simulink model "TST_PIntkVUs_DD"  (R2016b)
settings: Solver=FixedStepDiscrete  StartTime=0.0  StopTime=simTime  FixedStep=sampleTime  RelTol=1e-3
values from neighbouring files (symbols this model uses):
  testCase = 1    [initTST_PIntkVUs_DD_001.m]    (also in initTST_PIntkVUs_DD_002.m = 2; initTST_PIntkVUs_DD_003.m = 3; initTST_PIntkVUs_DD_004.m = 4; initTST_PIntkVUs_DD_005.m = 5)
libraries: UnitTest_Lib x98, simulink x8
(part 2 of 3)

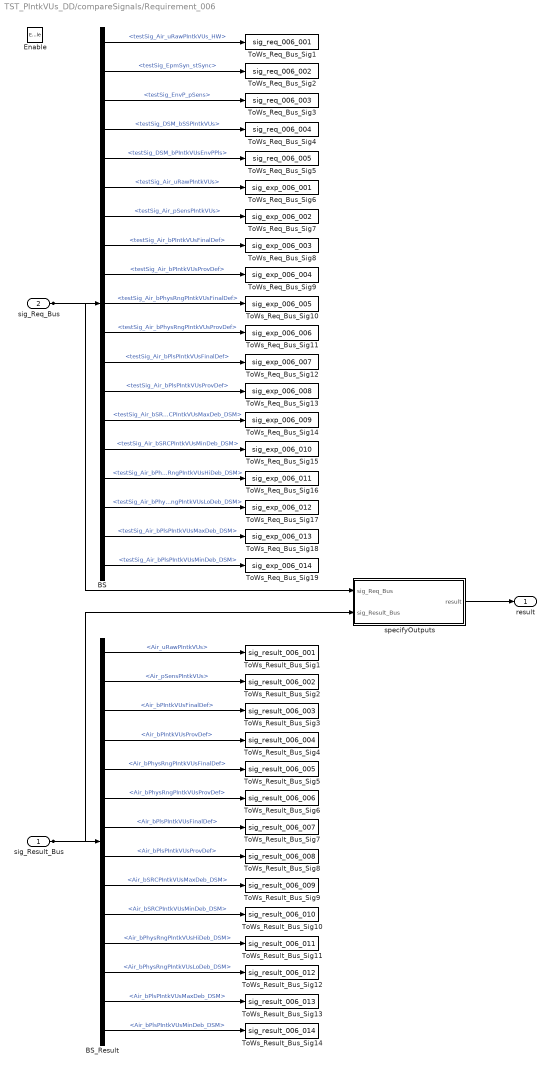
== system TST_PIntkVUs_DD/compareSignals/Requirement_006 ==
  sig_Result_Bus : Inport
  sig_Req_Bus : Inport  Port=2
  Enable : EnablePort
  BS : BusSelector  OutputSignals=testSig_Air_uRawPIntkVUs_HW,testSig_EpmSyn_stSync,testSig_EnvP_pSens,testSig_DSM_bSSPIntkVUs,testSig_DSM_bPIntkVUsEnvPPls,testSig_Air_uRawPIntkVUs,testSig_Air_pSensPIntkVUs,testSig_Air_bPIntkVUsFinalDef,testSig_Air_bPIntkVUsProvDef,testSig_Air_bPhysRngPIntkVUsFinalDef,testSig_Air_bPhysRngPIntkVUsProvDef,testSig_Air_bPlsPIntkVUsFinalDef,testSig_Air_bPlsPIntkVUsProvDef,testSig_Air_bSRCPIntkVUsMaxDeb_DSM,testSig_Air_bSRCPIntkVUsMinDeb_DSM,testSig_Air_bPhysRngPIntkVUsHiDeb_DSM,testSig_Air_bPhysRngPIntkVUsLoDeb_DSM,testSig_Air_bPlsPIntkVUsMaxDeb_DSM,testSig_Air_bPlsPIntkVUsMinDeb_DSM
  BS_Result : BusSelector  OutputSignals=Air_uRawPIntkVUs,Air_pSensPIntkVUs,Air_bPIntkVUsFinalDef,Air_bPIntkVUsProvDef,Air_bPhysRngPIntkVUsFinalDef,Air_bPhysRngPIntkVUsProvDef,Air_bPlsPIntkVUsFinalDef,Air_bPlsPIntkVUsProvDef,Air_bSRCPIntkVUsMaxDeb_DSM,Air_bSRCPIntkVUsMinDeb_DSM,Air_bPhysRngPIntkVUsHiDeb_DSM,Air_bPhysRngPIntkVUsLoDeb_DSM,Air_bPlsPIntkVUsMaxDeb_DSM,Air_bPlsPIntkVUsMinDeb_DSM
  ToWs_Req_Bus_Sig1 : ToWorkspace  VariableName=sig_req_006_001  SaveFormat=Structure With Time
  ToWs_Req_Bus_Sig10 : ToWorkspace  VariableName=sig_exp_006_005  SaveFormat=Structure With Time
  ToWs_Req_Bus_Sig11 : ToWorkspace  VariableName=sig_exp_006_006  SaveFormat=Structure With Time
  ToWs_Req_Bus_Sig12 : ToWorkspace  VariableName=sig_exp_006_007  SaveFormat=Structure With Time
  ToWs_Req_Bus_Sig13 : ToWorkspace  VariableName=sig_exp_006_008  SaveFormat=Structure With Time
  ToWs_Req_Bus_Sig14 : ToWorkspace  VariableName=sig_exp_006_009  SaveFormat=Structure With Time
  ToWs_Req_Bus_Sig15 : ToWorkspace  VariableName=sig_exp_006_010  SaveFormat=Structure With Time
  ToWs_Req_Bus_Sig16 : ToWorkspace  VariableName=sig_exp_006_011  SaveFormat=Structure With Time
  ToWs_Req_Bus_Sig17 : ToWorkspace  VariableName=sig_exp_006_012  SaveFormat=Structure With Time
  ToWs_Req_Bus_Sig18 : ToWorkspace  VariableName=sig_exp_006_013  SaveFormat=Structure With Time
  ToWs_Req_Bus_Sig19 : ToWorkspace  VariableName=sig_exp_006_014  SaveFormat=Structure With Time
  ToWs_Req_Bus_Sig2 : ToWorkspace  VariableName=sig_req_006_002  SaveFormat=Structure With Time
  ToWs_Req_Bus_Sig3 : ToWorkspace  VariableName=sig_req_006_003  SaveFormat=Structure With Time
  ToWs_Req_Bus_Sig4 : ToWorkspace  VariableName=sig_req_006_004  SaveFormat=Structure With Time
  ToWs_Req_Bus_Sig5 : ToWorkspace  VariableName=sig_req_006_005  SaveFormat=Structure With Time
  ToWs_Req_Bus_Sig6 : ToWorkspace  VariableName=sig_exp_006_001  SaveFormat=Structure With Time
  ToWs_Req_Bus_Sig7 : ToWorkspace  VariableName=sig_exp_006_002  SaveFormat=Structure With Time
  ToWs_Req_Bus_Sig8 : ToWorkspace  VariableName=sig_exp_006_003  SaveFormat=Structure With Time
  ToWs_Req_Bus_Sig9 : ToWorkspace  VariableName=sig_exp_006_004  SaveFormat=Structure With Time
  ToWs_Result_Bus_Sig1 : ToWorkspace  VariableName=sig_result_006_001  SaveFormat=Structure With Time
  ToWs_Result_Bus_Sig10 : ToWorkspace  VariableName=sig_result_006_010  SaveFormat=Structure With Time
  ToWs_Result_Bus_Sig11 : ToWorkspace  VariableName=sig_result_006_011  SaveFormat=Structure With Time
  ToWs_Result_Bus_Sig12 : ToWorkspace  VariableName=sig_result_006_012  SaveFormat=Structure With Time
  ToWs_Result_Bus_Sig13 : ToWorkspace  VariableName=sig_result_006_013  SaveFormat=Structure With Time
  ToWs_Result_Bus_Sig14 : ToWorkspace  VariableName=sig_result_006_014  SaveFormat=Structure With Time
  ToWs_Result_Bus_Sig2 : ToWorkspace  VariableName=sig_result_006_002  SaveFormat=Structure With Time
  ToWs_Result_Bus_Sig3 : ToWorkspace  VariableName=sig_result_006_003  SaveFormat=Structure With Time
  ToWs_Result_Bus_Sig4 : ToWorkspace  VariableName=sig_result_006_004  SaveFormat=Structure With Time
  ToWs_Result_Bus_Sig5 : ToWorkspace  VariableName=sig_result_006_005  SaveFormat=Structure With Time
  ToWs_Result_Bus_Sig6 : ToWorkspace  VariableName=sig_result_006_006  SaveFormat=Structure With Time
  ToWs_Result_Bus_Sig7 : ToWorkspace  VariableName=sig_result_006_007  SaveFormat=Structure With Time
  ToWs_Result_Bus_Sig8 : ToWorkspace  VariableName=sig_result_006_008  SaveFormat=Structure With Time
  ToWs_Result_Bus_Sig9 : ToWorkspace  VariableName=sig_result_006_009  SaveFormat=Structure With Time
  specifyOutputs : Subsystem
  result : Outport
  wires:
  sig_Req_Bus/1 -> BS/1, specifyOutputs/1(sig_Req_Bus)
  BS/1 -> ToWs_Req_Bus_Sig1/1  "<testSig_Air_uRawPIntkVUs_HW>"
  BS/2 -> ToWs_Req_Bus_Sig2/1  "<testSig_EpmSyn_stSync>"
  BS/3 -> ToWs_Req_Bus_Sig3/1  "<testSig_EnvP_pSens>"
  BS/4 -> ToWs_Req_Bus_Sig4/1  "<testSig_DSM_bSSPIntkVUs>"
  BS/5 -> ToWs_Req_Bus_Sig5/1  "<testSig_DSM_bPIntkVUsEnvPPls>"
  BS/6 -> ToWs_Req_Bus_Sig6/1  "<testSig_Air_uRawPIntkVUs>"
  BS/7 -> ToWs_Req_Bus_Sig7/1  "<testSig_Air_pSensPIntkVUs>"
  BS/8 -> ToWs_Req_Bus_Sig8/1  "<testSig_Air_bPIntkVUsFinalDef>"
  BS/9 -> ToWs_Req_Bus_Sig9/1  "<testSig_Air_bPIntkVUsProvDef>"
  BS/10 -> ToWs_Req_Bus_Sig10/1  "<testSig_Air_bPhysRngPIntkVUsFinalDef>"
  BS/11 -> ToWs_Req_Bus_Sig11/1  "<testSig_Air_bPhysRngPIntkVUsProvDef>"
  BS/12 -> ToWs_Req_Bus_Sig12/1  "<testSig_Air_bPlsPIntkVUsFinalDef>"
  BS/13 -> ToWs_Req_Bus_Sig13/1  "<testSig_Air_bPlsPIntkVUsProvDef>"
  BS/14 -> ToWs_Req_Bus_Sig14/1  "<testSig_Air_bSRCPIntkVUsMaxDeb_DSM>"
  BS/15 -> ToWs_Req_Bus_Sig15/1  "<testSig_Air_bSRCPIntkVUsMinDeb_DSM>"
  BS/16 -> ToWs_Req_Bus_Sig16/1  "<testSig_Air_bPhysRngPIntkVUsHiDeb_DSM>"
  BS/17 -> ToWs_Req_Bus_Sig17/1  "<testSig_Air_bPhysRngPIntkVUsLoDeb_DSM>"
  BS/18 -> ToWs_Req_Bus_Sig18/1  "<testSig_Air_bPlsPIntkVUsMaxDeb_DSM>"
  BS/19 -> ToWs_Req_Bus_Sig19/1  "<testSig_Air_bPlsPIntkVUsMinDeb_DSM>"
  sig_Result_Bus/1 -> BS_Result/1, specifyOutputs/2(sig_Result_Bus)
  BS_Result/1 -> ToWs_Result_Bus_Sig1/1  "<Air_uRawPIntkVUs>"
  BS_Result/2 -> ToWs_Result_Bus_Sig2/1  "<Air_pSensPIntkVUs>"
  BS_Result/3 -> ToWs_Result_Bus_Sig3/1  "<Air_bPIntkVUsFinalDef>"
  BS_Result/4 -> ToWs_Result_Bus_Sig4/1  "<Air_bPIntkVUsProvDef>"
  BS_Result/5 -> ToWs_Result_Bus_Sig5/1  "<Air_bPhysRngPIntkVUsFinalDef>"
  BS_Result/6 -> ToWs_Result_Bus_Sig6/1  "<Air_bPhysRngPIntkVUsProvDef>"
  BS_Result/7 -> ToWs_Result_Bus_Sig7/1  "<Air_bPlsPIntkVUsFinalDef>"
  BS_Result/8 -> ToWs_Result_Bus_Sig8/1  "<Air_bPlsPIntkVUsProvDef>"
  BS_Result/9 -> ToWs_Result_Bus_Sig9/1  "<Air_bSRCPIntkVUsMaxDeb_DSM>"
  BS_Result/10 -> ToWs_Result_Bus_Sig10/1  "<Air_bSRCPIntkVUsMinDeb_DSM>"
  BS_Result/11 -> ToWs_Result_Bus_Sig11/1  "<Air_bPhysRngPIntkVUsHiDeb_DSM>"
  BS_Result/12 -> ToWs_Result_Bus_Sig12/1  "<Air_bPhysRngPIntkVUsLoDeb_DSM>"
  BS_Result/13 -> ToWs_Result_Bus_Sig13/1  "<Air_bPlsPIntkVUsMaxDeb_DSM>"
  BS_Result/14 -> ToWs_Result_Bus_Sig14/1  "<Air_bPlsPIntkVUsMinDeb_DSM>"
  specifyOutputs/1(result) -> result/1

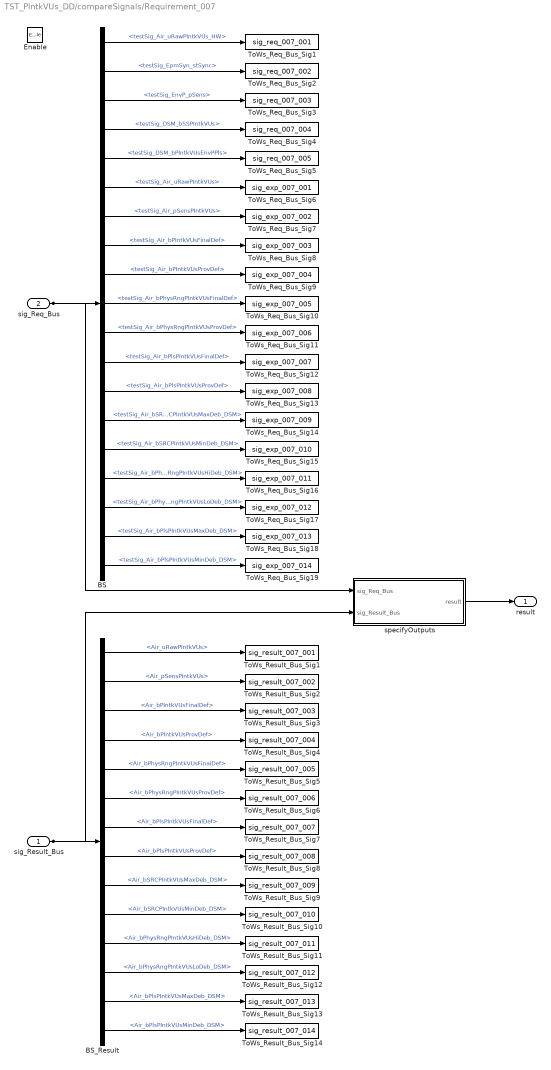
== system TST_PIntkVUs_DD/compareSignals/Requirement_007 ==
  sig_Result_Bus : Inport
  sig_Req_Bus : Inport  Port=2
  Enable : EnablePort
  BS : BusSelector  OutputSignals=testSig_Air_uRawPIntkVUs_HW,testSig_EpmSyn_stSync,testSig_EnvP_pSens,testSig_DSM_bSSPIntkVUs,testSig_DSM_bPIntkVUsEnvPPls,testSig_Air_uRawPIntkVUs,testSig_Air_pSensPIntkVUs,testSig_Air_bPIntkVUsFinalDef,testSig_Air_bPIntkVUsProvDef,testSig_Air_bPhysRngPIntkVUsFinalDef,testSig_Air_bPhysRngPIntkVUsProvDef,testSig_Air_bPlsPIntkVUsFinalDef,testSig_Air_bPlsPIntkVUsProvDef,testSig_Air_bSRCPIntkVUsMaxDeb_DSM,testSig_Air_bSRCPIntkVUsMinDeb_DSM,testSig_Air_bPhysRngPIntkVUsHiDeb_DSM,testSig_Air_bPhysRngPIntkVUsLoDeb_DSM,testSig_Air_bPlsPIntkVUsMaxDeb_DSM,testSig_Air_bPlsPIntkVUsMinDeb_DSM
  BS_Result : BusSelector  OutputSignals=Air_uRawPIntkVUs,Air_pSensPIntkVUs,Air_bPIntkVUsFinalDef,Air_bPIntkVUsProvDef,Air_bPhysRngPIntkVUsFinalDef,Air_bPhysRngPIntkVUsProvDef,Air_bPlsPIntkVUsFinalDef,Air_bPlsPIntkVUsProvDef,Air_bSRCPIntkVUsMaxDeb_DSM,Air_bSRCPIntkVUsMinDeb_DSM,Air_bPhysRngPIntkVUsHiDeb_DSM,Air_bPhysRngPIntkVUsLoDeb_DSM,Air_bPlsPIntkVUsMaxDeb_DSM,Air_bPlsPIntkVUsMinDeb_DSM
  ToWs_Req_Bus_Sig1 : ToWorkspace  VariableName=sig_req_007_001  SaveFormat=Structure With Time
  ToWs_Req_Bus_Sig10 : ToWorkspace  VariableName=sig_exp_007_005  SaveFormat=Structure With Time
  ToWs_Req_Bus_Sig11 : ToWorkspace  VariableName=sig_exp_007_006  SaveFormat=Structure With Time
  ToWs_Req_Bus_Sig12 : ToWorkspace  VariableName=sig_exp_007_007  SaveFormat=Structure With Time
  ToWs_Req_Bus_Sig13 : ToWorkspace  VariableName=sig_exp_007_008  SaveFormat=Structure With Time
  ToWs_Req_Bus_Sig14 : ToWorkspace  VariableName=sig_exp_007_009  SaveFormat=Structure With Time
  ToWs_Req_Bus_Sig15 : ToWorkspace  VariableName=sig_exp_007_010  SaveFormat=Structure With Time
  ToWs_Req_Bus_Sig16 : ToWorkspace  VariableName=sig_exp_007_011  SaveFormat=Structure With Time
  ToWs_Req_Bus_Sig17 : ToWorkspace  VariableName=sig_exp_007_012  SaveFormat=Structure With Time
  ToWs_Req_Bus_Sig18 : ToWorkspace  VariableName=sig_exp_007_013  SaveFormat=Structure With Time
  ToWs_Req_Bus_Sig19 : ToWorkspace  VariableName=sig_exp_007_014  SaveFormat=Structure With Time
  ToWs_Req_Bus_Sig2 : ToWorkspace  VariableName=sig_req_007_002  SaveFormat=Structure With Time
  ToWs_Req_Bus_Sig3 : ToWorkspace  VariableName=sig_req_007_003  SaveFormat=Structure With Time
  ToWs_Req_Bus_Sig4 : ToWorkspace  VariableName=sig_req_007_004  SaveFormat=Structure With Time
  ToWs_Req_Bus_Sig5 : ToWorkspace  VariableName=sig_req_007_005  SaveFormat=Structure With Time
  ToWs_Req_Bus_Sig6 : ToWorkspace  VariableName=sig_exp_007_001  SaveFormat=Structure With Time
  ToWs_Req_Bus_Sig7 : ToWorkspace  VariableName=sig_exp_007_002  SaveFormat=Structure With Time
  ToWs_Req_Bus_Sig8 : ToWorkspace  VariableName=sig_exp_007_003  SaveFormat=Structure With Time
  ToWs_Req_Bus_Sig9 : ToWorkspace  VariableName=sig_exp_007_004  SaveFormat=Structure With Time
  ToWs_Result_Bus_Sig1 : ToWorkspace  VariableName=sig_result_007_001  SaveFormat=Structure With Time
  ToWs_Result_Bus_Sig10 : ToWorkspace  VariableName=sig_result_007_010  SaveFormat=Structure With Time
  ToWs_Result_Bus_Sig11 : ToWorkspace  VariableName=sig_result_007_011  SaveFormat=Structure With Time
  ToWs_Result_Bus_Sig12 : ToWorkspace  VariableName=sig_result_007_012  SaveFormat=Structure With Time
  ToWs_Result_Bus_Sig13 : ToWorkspace  VariableName=sig_result_007_013  SaveFormat=Structure With Time
  ToWs_Result_Bus_Sig14 : ToWorkspace  VariableName=sig_result_007_014  SaveFormat=Structure With Time
  ToWs_Result_Bus_Sig2 : ToWorkspace  VariableName=sig_result_007_002  SaveFormat=Structure With Time
  ToWs_Result_Bus_Sig3 : ToWorkspace  VariableName=sig_result_007_003  SaveFormat=Structure With Time
  ToWs_Result_Bus_Sig4 : ToWorkspace  VariableName=sig_result_007_004  SaveFormat=Structure With Time
  ToWs_Result_Bus_Sig5 : ToWorkspace  VariableName=sig_result_007_005  SaveFormat=Structure With Time
  ToWs_Result_Bus_Sig6 : ToWorkspace  VariableName=sig_result_007_006  SaveFormat=Structure With Time
  ToWs_Result_Bus_Sig7 : ToWorkspace  VariableName=sig_result_007_007  SaveFormat=Structure With Time
  ToWs_Result_Bus_Sig8 : ToWorkspace  VariableName=sig_result_007_008  SaveFormat=Structure With Time
  ToWs_Result_Bus_Sig9 : ToWorkspace  VariableName=sig_result_007_009  SaveFormat=Structure With Time
  specifyOutputs : Subsystem
  result : Outport
  wires:
  sig_Req_Bus/1 -> BS/1, specifyOutputs/1(sig_Req_Bus)
  BS/1 -> ToWs_Req_Bus_Sig1/1  "<testSig_Air_uRawPIntkVUs_HW>"
  BS/2 -> ToWs_Req_Bus_Sig2/1  "<testSig_EpmSyn_stSync>"
  BS/3 -> ToWs_Req_Bus_Sig3/1  "<testSig_EnvP_pSens>"
  BS/4 -> ToWs_Req_Bus_Sig4/1  "<testSig_DSM_bSSPIntkVUs>"
  BS/5 -> ToWs_Req_Bus_Sig5/1  "<testSig_DSM_bPIntkVUsEnvPPls>"
  BS/6 -> ToWs_Req_Bus_Sig6/1  "<testSig_Air_uRawPIntkVUs>"
  BS/7 -> ToWs_Req_Bus_Sig7/1  "<testSig_Air_pSensPIntkVUs>"
  BS/8 -> ToWs_Req_Bus_Sig8/1  "<testSig_Air_bPIntkVUsFinalDef>"
  BS/9 -> ToWs_Req_Bus_Sig9/1  "<testSig_Air_bPIntkVUsProvDef>"
  BS/10 -> ToWs_Req_Bus_Sig10/1  "<testSig_Air_bPhysRngPIntkVUsFinalDef>"
  BS/11 -> ToWs_Req_Bus_Sig11/1  "<testSig_Air_bPhysRngPIntkVUsProvDef>"
  BS/12 -> ToWs_Req_Bus_Sig12/1  "<testSig_Air_bPlsPIntkVUsFinalDef>"
  BS/13 -> ToWs_Req_Bus_Sig13/1  "<testSig_Air_bPlsPIntkVUsProvDef>"
  BS/14 -> ToWs_Req_Bus_Sig14/1  "<testSig_Air_bSRCPIntkVUsMaxDeb_DSM>"
  BS/15 -> ToWs_Req_Bus_Sig15/1  "<testSig_Air_bSRCPIntkVUsMinDeb_DSM>"
  BS/16 -> ToWs_Req_Bus_Sig16/1  "<testSig_Air_bPhysRngPIntkVUsHiDeb_DSM>"
  BS/17 -> ToWs_Req_Bus_Sig17/1  "<testSig_Air_bPhysRngPIntkVUsLoDeb_DSM>"
  BS/18 -> ToWs_Req_Bus_Sig18/1  "<testSig_Air_bPlsPIntkVUsMaxDeb_DSM>"
  BS/19 -> ToWs_Req_Bus_Sig19/1  "<testSig_Air_bPlsPIntkVUsMinDeb_DSM>"
  sig_Result_Bus/1 -> BS_Result/1, specifyOutputs/2(sig_Result_Bus)
  BS_Result/1 -> ToWs_Result_Bus_Sig1/1  "<Air_uRawPIntkVUs>"
  BS_Result/2 -> ToWs_Result_Bus_Sig2/1  "<Air_pSensPIntkVUs>"
  BS_Result/3 -> ToWs_Result_Bus_Sig3/1  "<Air_bPIntkVUsFinalDef>"
  BS_Result/4 -> ToWs_Result_Bus_Sig4/1  "<Air_bPIntkVUsProvDef>"
  BS_Result/5 -> ToWs_Result_Bus_Sig5/1  "<Air_bPhysRngPIntkVUsFinalDef>"
  BS_Result/6 -> ToWs_Result_Bus_Sig6/1  "<Air_bPhysRngPIntkVUsProvDef>"
  BS_Result/7 -> ToWs_Result_Bus_Sig7/1  "<Air_bPlsPIntkVUsFinalDef>"
  BS_Result/8 -> ToWs_Result_Bus_Sig8/1  "<Air_bPlsPIntkVUsProvDef>"
  BS_Result/9 -> ToWs_Result_Bus_Sig9/1  "<Air_bSRCPIntkVUsMaxDeb_DSM>"
  BS_Result/10 -> ToWs_Result_Bus_Sig10/1  "<Air_bSRCPIntkVUsMinDeb_DSM>"
  BS_Result/11 -> ToWs_Result_Bus_Sig11/1  "<Air_bPhysRngPIntkVUsHiDeb_DSM>"
  BS_Result/12 -> ToWs_Result_Bus_Sig12/1  "<Air_bPhysRngPIntkVUsLoDeb_DSM>"
  BS_Result/13 -> ToWs_Result_Bus_Sig13/1  "<Air_bPlsPIntkVUsMaxDeb_DSM>"
  BS_Result/14 -> ToWs_Result_Bus_Sig14/1  "<Air_bPlsPIntkVUsMinDeb_DSM>"
  specifyOutputs/1(result) -> result/1

== system TST_PIntkVUs_DD/simulationInput/testSignals_R001 ==
  BC : BusCreator  Inputs=19
  spec_Air_bPIntkVUsFinalDef : FromWorkspace  VariableName=testSig_Air_bPIntkVUsFinalDef  Interpolate=off  OutputAfterFinalValue=Holding final value
  spec_Air_bPIntkVUsProvDef : FromWorkspace  VariableName=testSig_Air_bPIntkVUsProvDef  Interpolate=off  OutputAfterFinalValue=Holding final value
  spec_Air_bPhysRngPIntkVUsFinalDef : FromWorkspace  VariableName=testSig_Air_bPhysRngPIntkVUsFinalDef  Interpolate=off  OutputAfterFinalValue=Holding final value
  spec_Air_bPhysRngPIntkVUsHiDeb_DSM : FromWorkspace  VariableName=testSig_Air_bPhysRngPIntkVUsHiDeb_DSM  Interpolate=off  OutputAfterFinalValue=Holding final value
  spec_Air_bPhysRngPIntkVUsLoDeb_DSM : FromWorkspace  VariableName=testSig_Air_bPhysRngPIntkVUsLoDeb_DSM  Interpolate=off  OutputAfterFinalValue=Holding final value
  spec_Air_bPhysRngPIntkVUsProvDef : FromWorkspace  VariableName=testSig_Air_bPhysRngPIntkVUsProvDef  Interpolate=off  OutputAfterFinalValue=Holding final value
  spec_Air_bPlsPIntkVUsFinalDef : FromWorkspace  VariableName=testSig_Air_bPlsPIntkVUsFinalDef  Interpolate=off  OutputAfterFinalValue=Holding final value
  spec_Air_bPlsPIntkVUsMaxDeb_DSM : FromWorkspace  VariableName=testSig_Air_bPlsPIntkVUsMaxDeb_DSM  Interpolate=off  OutputAfterFinalValue=Holding final value
  spec_Air_bPlsPIntkVUsMinDeb_DSM : FromWorkspace  VariableName=testSig_Air_bPlsPIntkVUsMinDeb_DSM  Interpolate=off  OutputAfterFinalValue=Holding final value
  spec_Air_bPlsPIntkVUsProvDef : FromWorkspace  VariableName=testSig_Air_bPlsPIntkVUsProvDef  Interpolate=off  OutputAfterFinalValue=Holding final value
  spec_Air_bSRCPIntkVUsMaxDeb_DSM : FromWorkspace  VariableName=testSig_Air_bSRCPIntkVUsMaxDeb_DSM  Interpolate=off  OutputAfterFinalValue=Holding final value
  spec_Air_bSRCPIntkVUsMinDeb_DSM : FromWorkspace  VariableName=testSig_Air_bSRCPIntkVUsMinDeb_DSM  Interpolate=off  OutputAfterFinalValue=Holding final value
  spec_Air_pSensPIntkVUs : FromWorkspace  VariableName=testSig_Air_pSensPIntkVUs  Interpolate=off  OutputAfterFinalValue=Holding final value
  spec_Air_uRawPIntkVUs : FromWorkspace  VariableName=testSig_Air_uRawPIntkVUs  Interpolate=off  OutputAfterFinalValue=Holding final value
  spec_Air_uRawPIntkVUs_HW : FromWorkspace  VariableName=testSig_Air_uRawPIntkVUs_HW  Interpolate=off  OutputAfterFinalValue=Holding final value
  spec_DSM_bPIntkVUsEnvPPls : FromWorkspace  VariableName=testSig_DSM_bPIntkVUsEnvPPls  Interpolate=off  OutputAfterFinalValue=Holding final value
  spec_DSM_bSSPIntkVUs : FromWorkspace  VariableName=testSig_DSM_bSSPIntkVUs  Interpolate=off  OutputAfterFinalValue=Holding final value
  spec_EnvP_pSens : FromWorkspace  VariableName=testSig_EnvP_pSens  Interpolate=off  OutputAfterFinalValue=Holding final value
  spec_EpmSyn_stSync : FromWorkspace  VariableName=testSig_EpmSyn_stSync  Interpolate=off  OutputAfterFinalValue=Holding final value
  testSignals : Outport
  wires:
  BC/1 -> testSignals/1
  spec_Air_uRawPIntkVUs_HW/1 -> BC/1  "testSig_Air_uRawPIntkVUs_HW"
  spec_EpmSyn_stSync/1 -> BC/2  "testSig_EpmSyn_stSync"
  spec_EnvP_pSens/1 -> BC/3  "testSig_EnvP_pSens"
  spec_DSM_bSSPIntkVUs/1 -> BC/4  "testSig_DSM_bSSPIntkVUs"
  spec_DSM_bPIntkVUsEnvPPls/1 -> BC/5  "testSig_DSM_bPIntkVUsEnvPPls"
  spec_Air_uRawPIntkVUs/1 -> BC/6  "testSig_Air_uRawPIntkVUs"
  spec_Air_pSensPIntkVUs/1 -> BC/7  "testSig_Air_pSensPIntkVUs"
  spec_Air_bPIntkVUsFinalDef/1 -> BC/8  "testSig_Air_bPIntkVUsFinalDef"
  spec_Air_bPIntkVUsProvDef/1 -> BC/9  "testSig_Air_bPIntkVUsProvDef"
  spec_Air_bPhysRngPIntkVUsFinalDef/1 -> BC/10  "testSig_Air_bPhysRngPIntkVUsFinalDef"
  spec_Air_bPhysRngPIntkVUsProvDef/1 -> BC/11  "testSig_Air_bPhysRngPIntkVUsProvDef"
  spec_Air_bPlsPIntkVUsFinalDef/1 -> BC/12  "testSig_Air_bPlsPIntkVUsFinalDef"
  spec_Air_bPlsPIntkVUsProvDef/1 -> BC/13  "testSig_Air_bPlsPIntkVUsProvDef"
  spec_Air_bSRCPIntkVUsMaxDeb_DSM/1 -> BC/14  "testSig_Air_bSRCPIntkVUsMaxDeb_DSM"
  spec_Air_bSRCPIntkVUsMinDeb_DSM/1 -> BC/15  "testSig_Air_bSRCPIntkVUsMinDeb_DSM"
  spec_Air_bPhysRngPIntkVUsHiDeb_DSM/1 -> BC/16  "testSig_Air_bPhysRngPIntkVUsHiDeb_DSM"
  spec_Air_bPhysRngPIntkVUsLoDeb_DSM/1 -> BC/17  "testSig_Air_bPhysRngPIntkVUsLoDeb_DSM"
  spec_Air_bPlsPIntkVUsMaxDeb_DSM/1 -> BC/18  "testSig_Air_bPlsPIntkVUsMaxDeb_DSM"
  spec_Air_bPlsPIntkVUsMinDeb_DSM/1 -> BC/19  "testSig_Air_bPlsPIntkVUsMinDeb_DSM"

== system TST_PIntkVUs_DD/simulationInput/testSignals_R002 ==
  BC : BusCreator  Inputs=19
  spec_Air_bPIntkVUsFinalDef : FromWorkspace  VariableName=testSig_Air_bPIntkVUsFinalDef  Interpolate=off  OutputAfterFinalValue=Holding final value
  spec_Air_bPIntkVUsProvDef : FromWorkspace  VariableName=testSig_Air_bPIntkVUsProvDef  Interpolate=off  OutputAfterFinalValue=Holding final value
  spec_Air_bPhysRngPIntkVUsFinalDef : FromWorkspace  VariableName=testSig_Air_bPhysRngPIntkVUsFinalDef  Interpolate=off  OutputAfterFinalValue=Holding final value
  spec_Air_bPhysRngPIntkVUsHiDeb_DSM : FromWorkspace  VariableName=testSig_Air_bPhysRngPIntkVUsHiDeb_DSM  Interpolate=off  OutputAfterFinalValue=Holding final value
  spec_Air_bPhysRngPIntkVUsLoDeb_DSM : FromWorkspace  VariableName=testSig_Air_bPhysRngPIntkVUsLoDeb_DSM  Interpolate=off  OutputAfterFinalValue=Holding final value
  spec_Air_bPhysRngPIntkVUsProvDef : FromWorkspace  VariableName=testSig_Air_bPhysRngPIntkVUsProvDef  Interpolate=off  OutputAfterFinalValue=Holding final value
  spec_Air_bPlsPIntkVUsFinalDef : FromWorkspace  VariableName=testSig_Air_bPlsPIntkVUsFinalDef  Interpolate=off  OutputAfterFinalValue=Holding final value
  spec_Air_bPlsPIntkVUsMaxDeb_DSM : FromWorkspace  VariableName=testSig_Air_bPlsPIntkVUsMaxDeb_DSM  Interpolate=off  OutputAfterFinalValue=Holding final value
  spec_Air_bPlsPIntkVUsMinDeb_DSM : FromWorkspace  VariableName=testSig_Air_bPlsPIntkVUsMinDeb_DSM  Interpolate=off  OutputAfterFinalValue=Holding final value
  spec_Air_bPlsPIntkVUsProvDef : FromWorkspace  VariableName=testSig_Air_bPlsPIntkVUsProvDef  Interpolate=off  OutputAfterFinalValue=Holding final value
  spec_Air_bSRCPIntkVUsMaxDeb_DSM : FromWorkspace  VariableName=testSig_Air_bSRCPIntkVUsMaxDeb_DSM  Interpolate=off  OutputAfterFinalValue=Holding final value
  spec_Air_bSRCPIntkVUsMinDeb_DSM : FromWorkspace  VariableName=testSig_Air_bSRCPIntkVUsMinDeb_DSM  Interpolate=off  OutputAfterFinalValue=Holding final value
  spec_Air_pSensPIntkVUs : FromWorkspace  VariableName=testSig_Air_pSensPIntkVUs  Interpolate=off  OutputAfterFinalValue=Holding final value
  spec_Air_uRawPIntkVUs : FromWorkspace  VariableName=testSig_Air_uRawPIntkVUs  Interpolate=off  OutputAfterFinalValue=Holding final value
  spec_Air_uRawPIntkVUs_HW : FromWorkspace  VariableName=testSig_Air_uRawPIntkVUs_HW  Interpolate=off  OutputAfterFinalValue=Holding final value
  spec_DSM_bPIntkVUsEnvPPls : FromWorkspace  VariableName=testSig_DSM_bPIntkVUsEnvPPls  Interpolate=off  OutputAfterFinalValue=Holding final value
  spec_DSM_bSSPIntkVUs : FromWorkspace  VariableName=testSig_DSM_bSSPIntkVUs  Interpolate=off  OutputAfterFinalValue=Holding final value
  spec_EnvP_pSens : FromWorkspace  VariableName=testSig_EnvP_pSens  Interpolate=off  OutputAfterFinalValue=Holding final value
  spec_EpmSyn_stSync : FromWorkspace  VariableName=testSig_EpmSyn_stSync  Interpolate=off  OutputAfterFinalValue=Holding final value
  testSignals : Outport
  wires:
  BC/1 -> testSignals/1
  spec_Air_uRawPIntkVUs_HW/1 -> BC/1  "testSig_Air_uRawPIntkVUs_HW"
  spec_EpmSyn_stSync/1 -> BC/2  "testSig_EpmSyn_stSync"
  spec_EnvP_pSens/1 -> BC/3  "testSig_EnvP_pSens"
  spec_DSM_bSSPIntkVUs/1 -> BC/4  "testSig_DSM_bSSPIntkVUs"
  spec_DSM_bPIntkVUsEnvPPls/1 -> BC/5  "testSig_DSM_bPIntkVUsEnvPPls"
  spec_Air_uRawPIntkVUs/1 -> BC/6  "testSig_Air_uRawPIntkVUs"
  spec_Air_pSensPIntkVUs/1 -> BC/7  "testSig_Air_pSensPIntkVUs"
  spec_Air_bPIntkVUsFinalDef/1 -> BC/8  "testSig_Air_bPIntkVUsFinalDef"
  spec_Air_bPIntkVUsProvDef/1 -> BC/9  "testSig_Air_bPIntkVUsProvDef"
  spec_Air_bPhysRngPIntkVUsFinalDef/1 -> BC/10  "testSig_Air_bPhysRngPIntkVUsFinalDef"
  spec_Air_bPhysRngPIntkVUsProvDef/1 -> BC/11  "testSig_Air_bPhysRngPIntkVUsProvDef"
  spec_Air_bPlsPIntkVUsFinalDef/1 -> BC/12  "testSig_Air_bPlsPIntkVUsFinalDef"
  spec_Air_bPlsPIntkVUsProvDef/1 -> BC/13  "testSig_Air_bPlsPIntkVUsProvDef"
  spec_Air_bSRCPIntkVUsMaxDeb_DSM/1 -> BC/14  "testSig_Air_bSRCPIntkVUsMaxDeb_DSM"
  spec_Air_bSRCPIntkVUsMinDeb_DSM/1 -> BC/15  "testSig_Air_bSRCPIntkVUsMinDeb_DSM"
  spec_Air_bPhysRngPIntkVUsHiDeb_DSM/1 -> BC/16  "testSig_Air_bPhysRngPIntkVUsHiDeb_DSM"
  spec_Air_bPhysRngPIntkVUsLoDeb_DSM/1 -> BC/17  "testSig_Air_bPhysRngPIntkVUsLoDeb_DSM"
  spec_Air_bPlsPIntkVUsMaxDeb_DSM/1 -> BC/18  "testSig_Air_bPlsPIntkVUsMaxDeb_DSM"
  spec_Air_bPlsPIntkVUsMinDeb_DSM/1 -> BC/19  "testSig_Air_bPlsPIntkVUsMinDeb_DSM"

== system TST_PIntkVUs_DD/simulationInput/testSignals_R003 ==
  BC : BusCreator  Inputs=19
  spec_Air_bPIntkVUsFinalDef : FromWorkspace  VariableName=testSig_Air_bPIntkVUsFinalDef  Interpolate=off  OutputAfterFinalValue=Holding final value
  spec_Air_bPIntkVUsProvDef : FromWorkspace  VariableName=testSig_Air_bPIntkVUsProvDef  Interpolate=off  OutputAfterFinalValue=Holding final value
  spec_Air_bPhysRngPIntkVUsFinalDef : FromWorkspace  VariableName=testSig_Air_bPhysRngPIntkVUsFinalDef  Interpolate=off  OutputAfterFinalValue=Holding final value
  spec_Air_bPhysRngPIntkVUsHiDeb_DSM : FromWorkspace  VariableName=testSig_Air_bPhysRngPIntkVUsHiDeb_DSM  Interpolate=off  OutputAfterFinalValue=Holding final value
  spec_Air_bPhysRngPIntkVUsLoDeb_DSM : FromWorkspace  VariableName=testSig_Air_bPhysRngPIntkVUsLoDeb_DSM  Interpolate=off  OutputAfterFinalValue=Holding final value
  spec_Air_bPhysRngPIntkVUsProvDef : FromWorkspace  VariableName=testSig_Air_bPhysRngPIntkVUsProvDef  Interpolate=off  OutputAfterFinalValue=Holding final value
  spec_Air_bPlsPIntkVUsFinalDef : FromWorkspace  VariableName=testSig_Air_bPlsPIntkVUsFinalDef  Interpolate=off  OutputAfterFinalValue=Holding final value
  spec_Air_bPlsPIntkVUsMaxDeb_DSM : FromWorkspace  VariableName=testSig_Air_bPlsPIntkVUsMaxDeb_DSM  Interpolate=off  OutputAfterFinalValue=Holding final value
  spec_Air_bPlsPIntkVUsMinDeb_DSM : FromWorkspace  VariableName=testSig_Air_bPlsPIntkVUsMinDeb_DSM  Interpolate=off  OutputAfterFinalValue=Holding final value
  spec_Air_bPlsPIntkVUsProvDef : FromWorkspace  VariableName=testSig_Air_bPlsPIntkVUsProvDef  Interpolate=off  OutputAfterFinalValue=Holding final value
  spec_Air_bSRCPIntkVUsMaxDeb_DSM : FromWorkspace  VariableName=testSig_Air_bSRCPIntkVUsMaxDeb_DSM  Interpolate=off  OutputAfterFinalValue=Holding final value
  spec_Air_bSRCPIntkVUsMinDeb_DSM : FromWorkspace  VariableName=testSig_Air_bSRCPIntkVUsMinDeb_DSM  Interpolate=off  OutputAfterFinalValue=Holding final value
  spec_Air_pSensPIntkVUs : FromWorkspace  VariableName=testSig_Air_pSensPIntkVUs  Interpolate=off  OutputAfterFinalValue=Holding final value
  spec_Air_uRawPIntkVUs : FromWorkspace  VariableName=testSig_Air_uRawPIntkVUs  Interpolate=off  OutputAfterFinalValue=Holding final value
  spec_Air_uRawPIntkVUs_HW : FromWorkspace  VariableName=testSig_Air_uRawPIntkVUs_HW  Interpolate=off  OutputAfterFinalValue=Holding final value
  spec_DSM_bPIntkVUsEnvPPls : FromWorkspace  VariableName=testSig_DSM_bPIntkVUsEnvPPls  Interpolate=off  OutputAfterFinalValue=Holding final value
  spec_DSM_bSSPIntkVUs : FromWorkspace  VariableName=testSig_DSM_bSSPIntkVUs  Interpolate=off  OutputAfterFinalValue=Holding final value
  spec_EnvP_pSens : FromWorkspace  VariableName=testSig_EnvP_pSens  Interpolate=off  OutputAfterFinalValue=Holding final value
  spec_EpmSyn_stSync : FromWorkspace  VariableName=testSig_EpmSyn_stSync  Interpolate=off  OutputAfterFinalValue=Holding final value
  testSignals : Outport
  wires:
  BC/1 -> testSignals/1
  spec_Air_uRawPIntkVUs_HW/1 -> BC/1  "testSig_Air_uRawPIntkVUs_HW"
  spec_EpmSyn_stSync/1 -> BC/2  "testSig_EpmSyn_stSync"
  spec_EnvP_pSens/1 -> BC/3  "testSig_EnvP_pSens"
  spec_DSM_bSSPIntkVUs/1 -> BC/4  "testSig_DSM_bSSPIntkVUs"
  spec_DSM_bPIntkVUsEnvPPls/1 -> BC/5  "testSig_DSM_bPIntkVUsEnvPPls"
  spec_Air_uRawPIntkVUs/1 -> BC/6  "testSig_Air_uRawPIntkVUs"
  spec_Air_pSensPIntkVUs/1 -> BC/7  "testSig_Air_pSensPIntkVUs"
  spec_Air_bPIntkVUsFinalDef/1 -> BC/8  "testSig_Air_bPIntkVUsFinalDef"
  spec_Air_bPIntkVUsProvDef/1 -> BC/9  "testSig_Air_bPIntkVUsProvDef"
  spec_Air_bPhysRngPIntkVUsFinalDef/1 -> BC/10  "testSig_Air_bPhysRngPIntkVUsFinalDef"
  spec_Air_bPhysRngPIntkVUsProvDef/1 -> BC/11  "testSig_Air_bPhysRngPIntkVUsProvDef"
  spec_Air_bPlsPIntkVUsFinalDef/1 -> BC/12  "testSig_Air_bPlsPIntkVUsFinalDef"
  spec_Air_bPlsPIntkVUsProvDef/1 -> BC/13  "testSig_Air_bPlsPIntkVUsProvDef"
  spec_Air_bSRCPIntkVUsMaxDeb_DSM/1 -> BC/14  "testSig_Air_bSRCPIntkVUsMaxDeb_DSM"
  spec_Air_bSRCPIntkVUsMinDeb_DSM/1 -> BC/15  "testSig_Air_bSRCPIntkVUsMinDeb_DSM"
  spec_Air_bPhysRngPIntkVUsHiDeb_DSM/1 -> BC/16  "testSig_Air_bPhysRngPIntkVUsHiDeb_DSM"
  spec_Air_bPhysRngPIntkVUsLoDeb_DSM/1 -> BC/17  "testSig_Air_bPhysRngPIntkVUsLoDeb_DSM"
  spec_Air_bPlsPIntkVUsMaxDeb_DSM/1 -> BC/18  "testSig_Air_bPlsPIntkVUsMaxDeb_DSM"
  spec_Air_bPlsPIntkVUsMinDeb_DSM/1 -> BC/19  "testSig_Air_bPlsPIntkVUsMinDeb_DSM"

== system TST_PIntkVUs_DD/simulationInput/testSignals_R004 ==
  BC : BusCreator  Inputs=19
  spec_Air_bPIntkVUsFinalDef : FromWorkspace  VariableName=testSig_Air_bPIntkVUsFinalDef  Interpolate=off  OutputAfterFinalValue=Holding final value
  spec_Air_bPIntkVUsProvDef : FromWorkspace  VariableName=testSig_Air_bPIntkVUsProvDef  Interpolate=off  OutputAfterFinalValue=Holding final value
  spec_Air_bPhysRngPIntkVUsFinalDef : FromWorkspace  VariableName=testSig_Air_bPhysRngPIntkVUsFinalDef  Interpolate=off  OutputAfterFinalValue=Holding final value
  spec_Air_bPhysRngPIntkVUsHiDeb_DSM : FromWorkspace  VariableName=testSig_Air_bPhysRngPIntkVUsHiDeb_DSM  Interpolate=off  OutputAfterFinalValue=Holding final value
  spec_Air_bPhysRngPIntkVUsLoDeb_DSM : FromWorkspace  VariableName=testSig_Air_bPhysRngPIntkVUsLoDeb_DSM  Interpolate=off  OutputAfterFinalValue=Holding final value
  spec_Air_bPhysRngPIntkVUsProvDef : FromWorkspace  VariableName=testSig_Air_bPhysRngPIntkVUsProvDef  Interpolate=off  OutputAfterFinalValue=Holding final value
  spec_Air_bPlsPIntkVUsFinalDef : FromWorkspace  VariableName=testSig_Air_bPlsPIntkVUsFinalDef  Interpolate=off  OutputAfterFinalValue=Holding final value
  spec_Air_bPlsPIntkVUsMaxDeb_DSM : FromWorkspace  VariableName=testSig_Air_bPlsPIntkVUsMaxDeb_DSM  Interpolate=off  OutputAfterFinalValue=Holding final value
  spec_Air_bPlsPIntkVUsMinDeb_DSM : FromWorkspace  VariableName=testSig_Air_bPlsPIntkVUsMinDeb_DSM  Interpolate=off  OutputAfterFinalValue=Holding final value
  spec_Air_bPlsPIntkVUsProvDef : FromWorkspace  VariableName=testSig_Air_bPlsPIntkVUsProvDef  Interpolate=off  OutputAfterFinalValue=Holding final value
  spec_Air_bSRCPIntkVUsMaxDeb_DSM : FromWorkspace  VariableName=testSig_Air_bSRCPIntkVUsMaxDeb_DSM  Interpolate=off  OutputAfterFinalValue=Holding final value
  spec_Air_bSRCPIntkVUsMinDeb_DSM : FromWorkspace  VariableName=testSig_Air_bSRCPIntkVUsMinDeb_DSM  Interpolate=off  OutputAfterFinalValue=Holding final value
  spec_Air_pSensPIntkVUs : FromWorkspace  VariableName=testSig_Air_pSensPIntkVUs  Interpolate=off  OutputAfterFinalValue=Holding final value
  spec_Air_uRawPIntkVUs : FromWorkspace  VariableName=testSig_Air_uRawPIntkVUs  Interpolate=off  OutputAfterFinalValue=Holding final value
  spec_Air_uRawPIntkVUs_HW : FromWorkspace  VariableName=testSig_Air_uRawPIntkVUs_HW  Interpolate=off  OutputAfterFinalValue=Holding final value
  spec_DSM_bPIntkVUsEnvPPls : FromWorkspace  VariableName=testSig_DSM_bPIntkVUsEnvPPls  Interpolate=off  OutputAfterFinalValue=Holding final value
  spec_DSM_bSSPIntkVUs : FromWorkspace  VariableName=testSig_DSM_bSSPIntkVUs  Interpolate=off  OutputAfterFinalValue=Holding final value
  spec_EnvP_pSens : FromWorkspace  VariableName=testSig_EnvP_pSens  Interpolate=off  OutputAfterFinalValue=Holding final value
  spec_EpmSyn_stSync : FromWorkspace  VariableName=testSig_EpmSyn_stSync  Interpolate=off  OutputAfterFinalValue=Holding final value
  testSignals : Outport
  wires:
  BC/1 -> testSignals/1
  spec_Air_uRawPIntkVUs_HW/1 -> BC/1  "testSig_Air_uRawPIntkVUs_HW"
  spec_EpmSyn_stSync/1 -> BC/2  "testSig_EpmSyn_stSync"
  spec_EnvP_pSens/1 -> BC/3  "testSig_EnvP_pSens"
  spec_DSM_bSSPIntkVUs/1 -> BC/4  "testSig_DSM_bSSPIntkVUs"
  spec_DSM_bPIntkVUsEnvPPls/1 -> BC/5  "testSig_DSM_bPIntkVUsEnvPPls"
  spec_Air_uRawPIntkVUs/1 -> BC/6  "testSig_Air_uRawPIntkVUs"
  spec_Air_pSensPIntkVUs/1 -> BC/7  "testSig_Air_pSensPIntkVUs"
  spec_Air_bPIntkVUsFinalDef/1 -> BC/8  "testSig_Air_bPIntkVUsFinalDef"
  spec_Air_bPIntkVUsProvDef/1 -> BC/9  "testSig_Air_bPIntkVUsProvDef"
  spec_Air_bPhysRngPIntkVUsFinalDef/1 -> BC/10  "testSig_Air_bPhysRngPIntkVUsFinalDef"
  spec_Air_bPhysRngPIntkVUsProvDef/1 -> BC/11  "testSig_Air_bPhysRngPIntkVUsProvDef"
  spec_Air_bPlsPIntkVUsFinalDef/1 -> BC/12  "testSig_Air_bPlsPIntkVUsFinalDef"
  spec_Air_bPlsPIntkVUsProvDef/1 -> BC/13  "testSig_Air_bPlsPIntkVUsProvDef"
  spec_Air_bSRCPIntkVUsMaxDeb_DSM/1 -> BC/14  "testSig_Air_bSRCPIntkVUsMaxDeb_DSM"
  spec_Air_bSRCPIntkVUsMinDeb_DSM/1 -> BC/15  "testSig_Air_bSRCPIntkVUsMinDeb_DSM"
  spec_Air_bPhysRngPIntkVUsHiDeb_DSM/1 -> BC/16  "testSig_Air_bPhysRngPIntkVUsHiDeb_DSM"
  spec_Air_bPhysRngPIntkVUsLoDeb_DSM/1 -> BC/17  "testSig_Air_bPhysRngPIntkVUsLoDeb_DSM"
  spec_Air_bPlsPIntkVUsMaxDeb_DSM/1 -> BC/18  "testSig_Air_bPlsPIntkVUsMaxDeb_DSM"
  spec_Air_bPlsPIntkVUsMinDeb_DSM/1 -> BC/19  "testSig_Air_bPlsPIntkVUsMinDeb_DSM"

== system TST_PIntkVUs_DD/simulationInput/testSignals_R005 ==
  BC : BusCreator  Inputs=19
  spec_Air_bPIntkVUsFinalDef : FromWorkspace  VariableName=testSig_Air_bPIntkVUsFinalDef  Interpolate=off  OutputAfterFinalValue=Holding final value
  spec_Air_bPIntkVUsProvDef : FromWorkspace  VariableName=testSig_Air_bPIntkVUsProvDef  Interpolate=off  OutputAfterFinalValue=Holding final value
  spec_Air_bPhysRngPIntkVUsFinalDef : FromWorkspace  VariableName=testSig_Air_bPhysRngPIntkVUsFinalDef  Interpolate=off  OutputAfterFinalValue=Holding final value
  spec_Air_bPhysRngPIntkVUsHiDeb_DSM : FromWorkspace  VariableName=testSig_Air_bPhysRngPIntkVUsHiDeb_DSM  Interpolate=off  OutputAfterFinalValue=Holding final value
  spec_Air_bPhysRngPIntkVUsLoDeb_DSM : FromWorkspace  VariableName=testSig_Air_bPhysRngPIntkVUsLoDeb_DSM  Interpolate=off  OutputAfterFinalValue=Holding final value
  spec_Air_bPhysRngPIntkVUsProvDef : FromWorkspace  VariableName=testSig_Air_bPhysRngPIntkVUsProvDef  Interpolate=off  OutputAfterFinalValue=Holding final value
  spec_Air_bPlsPIntkVUsFinalDef : FromWorkspace  VariableName=testSig_Air_bPlsPIntkVUsFinalDef  Interpolate=off  OutputAfterFinalValue=Holding final value
  spec_Air_bPlsPIntkVUsMaxDeb_DSM : FromWorkspace  VariableName=testSig_Air_bPlsPIntkVUsMaxDeb_DSM  Interpolate=off  OutputAfterFinalValue=Holding final value
  spec_Air_bPlsPIntkVUsMinDeb_DSM : FromWorkspace  VariableName=testSig_Air_bPlsPIntkVUsMinDeb_DSM  Interpolate=off  OutputAfterFinalValue=Holding final value
  spec_Air_bPlsPIntkVUsProvDef : FromWorkspace  VariableName=testSig_Air_bPlsPIntkVUsProvDef  Interpolate=off  OutputAfterFinalValue=Holding final value
  spec_Air_bSRCPIntkVUsMaxDeb_DSM : FromWorkspace  VariableName=testSig_Air_bSRCPIntkVUsMaxDeb_DSM  Interpolate=off  OutputAfterFinalValue=Holding final value
  spec_Air_bSRCPIntkVUsMinDeb_DSM : FromWorkspace  VariableName=testSig_Air_bSRCPIntkVUsMinDeb_DSM  Interpolate=off  OutputAfterFinalValue=Holding final value
  spec_Air_pSensPIntkVUs : FromWorkspace  VariableName=testSig_Air_pSensPIntkVUs  Interpolate=off  OutputAfterFinalValue=Holding final value
  spec_Air_uRawPIntkVUs : FromWorkspace  VariableName=testSig_Air_uRawPIntkVUs  Interpolate=off  OutputAfterFinalValue=Holding final value
  spec_Air_uRawPIntkVUs_HW : FromWorkspace  VariableName=testSig_Air_uRawPIntkVUs_HW  Interpolate=off  OutputAfterFinalValue=Holding final value
  spec_DSM_bPIntkVUsEnvPPls : FromWorkspace  VariableName=testSig_DSM_bPIntkVUsEnvPPls  Interpolate=off  OutputAfterFinalValue=Holding final value
  spec_DSM_bSSPIntkVUs : FromWorkspace  VariableName=testSig_DSM_bSSPIntkVUs  Interpolate=off  OutputAfterFinalValue=Holding final value
  spec_EnvP_pSens : FromWorkspace  VariableName=testSig_EnvP_pSens  Interpolate=off  OutputAfterFinalValue=Holding final value
  spec_EpmSyn_stSync : FromWorkspace  VariableName=testSig_EpmSyn_stSync  Interpolate=off  OutputAfterFinalValue=Holding final value
  testSignals : Outport
  wires:
  BC/1 -> testSignals/1
  spec_Air_uRawPIntkVUs_HW/1 -> BC/1  "testSig_Air_uRawPIntkVUs_HW"
  spec_EpmSyn_stSync/1 -> BC/2  "testSig_EpmSyn_stSync"
  spec_EnvP_pSens/1 -> BC/3  "testSig_EnvP_pSens"
  spec_DSM_bSSPIntkVUs/1 -> BC/4  "testSig_DSM_bSSPIntkVUs"
  spec_DSM_bPIntkVUsEnvPPls/1 -> BC/5  "testSig_DSM_bPIntkVUsEnvPPls"
  spec_Air_uRawPIntkVUs/1 -> BC/6  "testSig_Air_uRawPIntkVUs"
  spec_Air_pSensPIntkVUs/1 -> BC/7  "testSig_Air_pSensPIntkVUs"
  spec_Air_bPIntkVUsFinalDef/1 -> BC/8  "testSig_Air_bPIntkVUsFinalDef"
  spec_Air_bPIntkVUsProvDef/1 -> BC/9  "testSig_Air_bPIntkVUsProvDef"
  spec_Air_bPhysRngPIntkVUsFinalDef/1 -> BC/10  "testSig_Air_bPhysRngPIntkVUsFinalDef"
  spec_Air_bPhysRngPIntkVUsProvDef/1 -> BC/11  "testSig_Air_bPhysRngPIntkVUsProvDef"
  spec_Air_bPlsPIntkVUsFinalDef/1 -> BC/12  "testSig_Air_bPlsPIntkVUsFinalDef"
  spec_Air_bPlsPIntkVUsProvDef/1 -> BC/13  "testSig_Air_bPlsPIntkVUsProvDef"
  spec_Air_bSRCPIntkVUsMaxDeb_DSM/1 -> BC/14  "testSig_Air_bSRCPIntkVUsMaxDeb_DSM"
  spec_Air_bSRCPIntkVUsMinDeb_DSM/1 -> BC/15  "testSig_Air_bSRCPIntkVUsMinDeb_DSM"
  spec_Air_bPhysRngPIntkVUsHiDeb_DSM/1 -> BC/16  "testSig_Air_bPhysRngPIntkVUsHiDeb_DSM"
  spec_Air_bPhysRngPIntkVUsLoDeb_DSM/1 -> BC/17  "testSig_Air_bPhysRngPIntkVUsLoDeb_DSM"
  spec_Air_bPlsPIntkVUsMaxDeb_DSM/1 -> BC/18  "testSig_Air_bPlsPIntkVUsMaxDeb_DSM"
  spec_Air_bPlsPIntkVUsMinDeb_DSM/1 -> BC/19  "testSig_Air_bPlsPIntkVUsMinDeb_DSM"

== system TST_PIntkVUs_DD/simulationInput/testSignals_R006 ==
  BC : BusCreator  Inputs=19
  spec_Air_bPIntkVUsFinalDef : FromWorkspace  VariableName=testSig_Air_bPIntkVUsFinalDef  Interpolate=off  OutputAfterFinalValue=Holding final value
  spec_Air_bPIntkVUsProvDef : FromWorkspace  VariableName=testSig_Air_bPIntkVUsProvDef  Interpolate=off  OutputAfterFinalValue=Holding final value
  spec_Air_bPhysRngPIntkVUsFinalDef : FromWorkspace  VariableName=testSig_Air_bPhysRngPIntkVUsFinalDef  Interpolate=off  OutputAfterFinalValue=Holding final value
  spec_Air_bPhysRngPIntkVUsHiDeb_DSM : FromWorkspace  VariableName=testSig_Air_bPhysRngPIntkVUsHiDeb_DSM  Interpolate=off  OutputAfterFinalValue=Holding final value
  spec_Air_bPhysRngPIntkVUsLoDeb_DSM : FromWorkspace  VariableName=testSig_Air_bPhysRngPIntkVUsLoDeb_DSM  Interpolate=off  OutputAfterFinalValue=Holding final value
  spec_Air_bPhysRngPIntkVUsProvDef : FromWorkspace  VariableName=testSig_Air_bPhysRngPIntkVUsProvDef  Interpolate=off  OutputAfterFinalValue=Holding final value
  spec_Air_bPlsPIntkVUsFinalDef : FromWorkspace  VariableName=testSig_Air_bPlsPIntkVUsFinalDef  Interpolate=off  OutputAfterFinalValue=Holding final value
  spec_Air_bPlsPIntkVUsMaxDeb_DSM : FromWorkspace  VariableName=testSig_Air_bPlsPIntkVUsMaxDeb_DSM  Interpolate=off  OutputAfterFinalValue=Holding final value
  spec_Air_bPlsPIntkVUsMinDeb_DSM : FromWorkspace  VariableName=testSig_Air_bPlsPIntkVUsMinDeb_DSM  Interpolate=off  OutputAfterFinalValue=Holding final value
  spec_Air_bPlsPIntkVUsProvDef : FromWorkspace  VariableName=testSig_Air_bPlsPIntkVUsProvDef  Interpolate=off  OutputAfterFinalValue=Holding final value
  spec_Air_bSRCPIntkVUsMaxDeb_DSM : FromWorkspace  VariableName=testSig_Air_bSRCPIntkVUsMaxDeb_DSM  Interpolate=off  OutputAfterFinalValue=Holding final value
  spec_Air_bSRCPIntkVUsMinDeb_DSM : FromWorkspace  VariableName=testSig_Air_bSRCPIntkVUsMinDeb_DSM  Interpolate=off  OutputAfterFinalValue=Holding final value
  spec_Air_pSensPIntkVUs : FromWorkspace  VariableName=testSig_Air_pSensPIntkVUs  Interpolate=off  OutputAfterFinalValue=Holding final value
  spec_Air_uRawPIntkVUs : FromWorkspace  VariableName=testSig_Air_uRawPIntkVUs  Interpolate=off  OutputAfterFinalValue=Holding final value
  spec_Air_uRawPIntkVUs_HW : FromWorkspace  VariableName=testSig_Air_uRawPIntkVUs_HW  Interpolate=off  OutputAfterFinalValue=Holding final value
  spec_DSM_bPIntkVUsEnvPPls : FromWorkspace  VariableName=testSig_DSM_bPIntkVUsEnvPPls  Interpolate=off  OutputAfterFinalValue=Holding final value
  spec_DSM_bSSPIntkVUs : FromWorkspace  VariableName=testSig_DSM_bSSPIntkVUs  Interpolate=off  OutputAfterFinalValue=Holding final value
  spec_EnvP_pSens : FromWorkspace  VariableName=testSig_EnvP_pSens  Interpolate=off  OutputAfterFinalValue=Holding final value
  spec_EpmSyn_stSync : FromWorkspace  VariableName=testSig_EpmSyn_stSync  Interpolate=off  OutputAfterFinalValue=Holding final value
  testSignals : Outport
  wires:
  BC/1 -> testSignals/1
  spec_Air_uRawPIntkVUs_HW/1 -> BC/1  "testSig_Air_uRawPIntkVUs_HW"
  spec_EpmSyn_stSync/1 -> BC/2  "testSig_EpmSyn_stSync"
  spec_EnvP_pSens/1 -> BC/3  "testSig_EnvP_pSens"
  spec_DSM_bSSPIntkVUs/1 -> BC/4  "testSig_DSM_bSSPIntkVUs"
  spec_DSM_bPIntkVUsEnvPPls/1 -> BC/5  "testSig_DSM_bPIntkVUsEnvPPls"
  spec_Air_uRawPIntkVUs/1 -> BC/6  "testSig_Air_uRawPIntkVUs"
  spec_Air_pSensPIntkVUs/1 -> BC/7  "testSig_Air_pSensPIntkVUs"
  spec_Air_bPIntkVUsFinalDef/1 -> BC/8  "testSig_Air_bPIntkVUsFinalDef"
  spec_Air_bPIntkVUsProvDef/1 -> BC/9  "testSig_Air_bPIntkVUsProvDef"
  spec_Air_bPhysRngPIntkVUsFinalDef/1 -> BC/10  "testSig_Air_bPhysRngPIntkVUsFinalDef"
  spec_Air_bPhysRngPIntkVUsProvDef/1 -> BC/11  "testSig_Air_bPhysRngPIntkVUsProvDef"
  spec_Air_bPlsPIntkVUsFinalDef/1 -> BC/12  "testSig_Air_bPlsPIntkVUsFinalDef"
  spec_Air_bPlsPIntkVUsProvDef/1 -> BC/13  "testSig_Air_bPlsPIntkVUsProvDef"
  spec_Air_bSRCPIntkVUsMaxDeb_DSM/1 -> BC/14  "testSig_Air_bSRCPIntkVUsMaxDeb_DSM"
  spec_Air_bSRCPIntkVUsMinDeb_DSM/1 -> BC/15  "testSig_Air_bSRCPIntkVUsMinDeb_DSM"
  spec_Air_bPhysRngPIntkVUsHiDeb_DSM/1 -> BC/16  "testSig_Air_bPhysRngPIntkVUsHiDeb_DSM"
  spec_Air_bPhysRngPIntkVUsLoDeb_DSM/1 -> BC/17  "testSig_Air_bPhysRngPIntkVUsLoDeb_DSM"
  spec_Air_bPlsPIntkVUsMaxDeb_DSM/1 -> BC/18  "testSig_Air_bPlsPIntkVUsMaxDeb_DSM"
  spec_Air_bPlsPIntkVUsMinDeb_DSM/1 -> BC/19  "testSig_Air_bPlsPIntkVUsMinDeb_DSM"

== system TST_PIntkVUs_DD/simulationInput/testSignals_R007 ==
  BC : BusCreator  Inputs=19
  spec_Air_bPIntkVUsFinalDef : FromWorkspace  VariableName=testSig_Air_bPIntkVUsFinalDef  Interpolate=off  OutputAfterFinalValue=Holding final value
  spec_Air_bPIntkVUsProvDef : FromWorkspace  VariableName=testSig_Air_bPIntkVUsProvDef  Interpolate=off  OutputAfterFinalValue=Holding final value
  spec_Air_bPhysRngPIntkVUsFinalDef : FromWorkspace  VariableName=testSig_Air_bPhysRngPIntkVUsFinalDef  Interpolate=off  OutputAfterFinalValue=Holding final value
  spec_Air_bPhysRngPIntkVUsHiDeb_DSM : FromWorkspace  VariableName=testSig_Air_bPhysRngPIntkVUsHiDeb_DSM  Interpolate=off  OutputAfterFinalValue=Holding final value
  spec_Air_bPhysRngPIntkVUsLoDeb_DSM : FromWorkspace  VariableName=testSig_Air_bPhysRngPIntkVUsLoDeb_DSM  Interpolate=off  OutputAfterFinalValue=Holding final value
  spec_Air_bPhysRngPIntkVUsProvDef : FromWorkspace  VariableName=testSig_Air_bPhysRngPIntkVUsProvDef  Interpolate=off  OutputAfterFinalValue=Holding final value
  spec_Air_bPlsPIntkVUsFinalDef : FromWorkspace  VariableName=testSig_Air_bPlsPIntkVUsFinalDef  Interpolate=off  OutputAfterFinalValue=Holding final value
  spec_Air_bPlsPIntkVUsMaxDeb_DSM : FromWorkspace  VariableName=testSig_Air_bPlsPIntkVUsMaxDeb_DSM  Interpolate=off  OutputAfterFinalValue=Holding final value
  spec_Air_bPlsPIntkVUsMinDeb_DSM : FromWorkspace  VariableName=testSig_Air_bPlsPIntkVUsMinDeb_DSM  Interpolate=off  OutputAfterFinalValue=Holding final value
  spec_Air_bPlsPIntkVUsProvDef : FromWorkspace  VariableName=testSig_Air_bPlsPIntkVUsProvDef  Interpolate=off  OutputAfterFinalValue=Holding final value
  spec_Air_bSRCPIntkVUsMaxDeb_DSM : FromWorkspace  VariableName=testSig_Air_bSRCPIntkVUsMaxDeb_DSM  Interpolate=off  OutputAfterFinalValue=Holding final value
  spec_Air_bSRCPIntkVUsMinDeb_DSM : FromWorkspace  VariableName=testSig_Air_bSRCPIntkVUsMinDeb_DSM  Interpolate=off  OutputAfterFinalValue=Holding final value
  spec_Air_pSensPIntkVUs : FromWorkspace  VariableName=testSig_Air_pSensPIntkVUs  Interpolate=off  OutputAfterFinalValue=Holding final value
  spec_Air_uRawPIntkVUs : FromWorkspace  VariableName=testSig_Air_uRawPIntkVUs  Interpolate=off  OutputAfterFinalValue=Holding final value
  spec_Air_uRawPIntkVUs_HW : FromWorkspace  VariableName=testSig_Air_uRawPIntkVUs_HW  Interpolate=off  OutputAfterFinalValue=Holding final value
  spec_DSM_bPIntkVUsEnvPPls : FromWorkspace  VariableName=testSig_DSM_bPIntkVUsEnvPPls  Interpolate=off  OutputAfterFinalValue=Holding final value
  spec_DSM_bSSPIntkVUs : FromWorkspace  VariableName=testSig_DSM_bSSPIntkVUs  Interpolate=off  OutputAfterFinalValue=Holding final value
  spec_EnvP_pSens : FromWorkspace  VariableName=testSig_EnvP_pSens  Interpolate=off  OutputAfterFinalValue=Holding final value
  spec_EpmSyn_stSync : FromWorkspace  VariableName=testSig_EpmSyn_stSync  Interpolate=off  OutputAfterFinalValue=Holding final value
  testSignals : Outport
  wires:
  BC/1 -> testSignals/1
  spec_Air_uRawPIntkVUs_HW/1 -> BC/1  "testSig_Air_uRawPIntkVUs_HW"
  spec_EpmSyn_stSync/1 -> BC/2  "testSig_EpmSyn_stSync"
  spec_EnvP_pSens/1 -> BC/3  "testSig_EnvP_pSens"
  spec_DSM_bSSPIntkVUs/1 -> BC/4  "testSig_DSM_bSSPIntkVUs"
  spec_DSM_bPIntkVUsEnvPPls/1 -> BC/5  "testSig_DSM_bPIntkVUsEnvPPls"
  spec_Air_uRawPIntkVUs/1 -> BC/6  "testSig_Air_uRawPIntkVUs"
  spec_Air_pSensPIntkVUs/1 -> BC/7  "testSig_Air_pSensPIntkVUs"
  spec_Air_bPIntkVUsFinalDef/1 -> BC/8  "testSig_Air_bPIntkVUsFinalDef"
  spec_Air_bPIntkVUsProvDef/1 -> BC/9  "testSig_Air_bPIntkVUsProvDef"
  spec_Air_bPhysRngPIntkVUsFinalDef/1 -> BC/10  "testSig_Air_bPhysRngPIntkVUsFinalDef"
  spec_Air_bPhysRngPIntkVUsProvDef/1 -> BC/11  "testSig_Air_bPhysRngPIntkVUsProvDef"
  spec_Air_bPlsPIntkVUsFinalDef/1 -> BC/12  "testSig_Air_bPlsPIntkVUsFinalDef"
  spec_Air_bPlsPIntkVUsProvDef/1 -> BC/13  "testSig_Air_bPlsPIntkVUsProvDef"
  spec_Air_bSRCPIntkVUsMaxDeb_DSM/1 -> BC/14  "testSig_Air_bSRCPIntkVUsMaxDeb_DSM"
  spec_Air_bSRCPIntkVUsMinDeb_DSM/1 -> BC/15  "testSig_Air_bSRCPIntkVUsMinDeb_DSM"
  spec_Air_bPhysRngPIntkVUsHiDeb_DSM/1 -> BC/16  "testSig_Air_bPhysRngPIntkVUsHiDeb_DSM"
  spec_Air_bPhysRngPIntkVUsLoDeb_DSM/1 -> BC/17  "testSig_Air_bPhysRngPIntkVUsLoDeb_DSM"
  spec_Air_bPlsPIntkVUsMaxDeb_DSM/1 -> BC/18  "testSig_Air_bPlsPIntkVUsMaxDeb_DSM"
  spec_Air_bPlsPIntkVUsMinDeb_DSM/1 -> BC/19  "testSig_Air_bPlsPIntkVUsMinDeb_DSM"

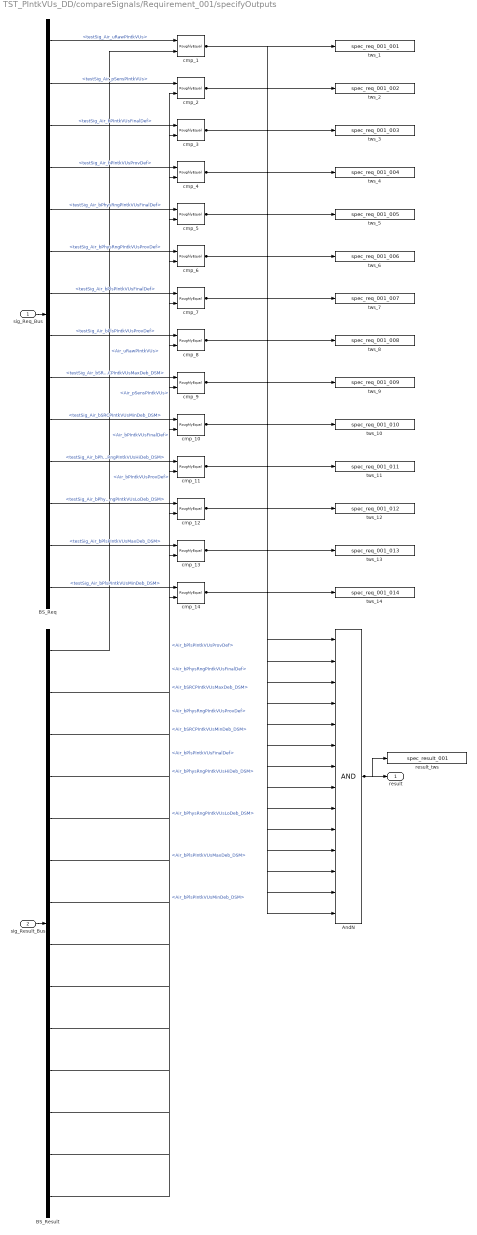
== system TST_PIntkVUs_DD/compareSignals/Requirement_001/specifyOutputs ==
  sig_Req_Bus : Inport
  sig_Result_Bus : Inport  Port=2
  AndN : Logic  Inputs=14
  BS_Req : BusSelector  OutputSignals=testSig_Air_uRawPIntkVUs,testSig_Air_pSensPIntkVUs,testSig_Air_bPIntkVUsFinalDef,testSig_Air_bPIntkVUsProvDef,testSig_Air_bPhysRngPIntkVUsFinalDef,testSig_Air_bPhysRngPIntkVUsProvDef,testSig_Air_bPlsPIntkVUsFinalDef,testSig_Air_bPlsPIntkVUsProvDef,testSig_Air_bSRCPIntkVUsMaxDeb_DSM,testSig_Air_bSRCPIntkVUsMinDeb_DSM,testSig_Air_bPhysRngPIntkVUsHiDeb_DSM,testSig_Air_bPhysRngPIntkVUsLoDeb_DSM,testSig_Air_bPlsPIntkVUsMaxDeb_DSM,testSig_Air_bPlsPIntkVUsMinDeb_DSM
  BS_Result : BusSelector  OutputSignals=Air_uRawPIntkVUs,Air_pSensPIntkVUs,Air_bPIntkVUsFinalDef,Air_bPIntkVUsProvDef,Air_bPhysRngPIntkVUsFinalDef,Air_bPhysRngPIntkVUsProvDef,Air_bPlsPIntkVUsFinalDef,Air_bPlsPIntkVUsProvDef,Air_bSRCPIntkVUsMaxDeb_DSM,Air_bSRCPIntkVUsMinDeb_DSM,Air_bPhysRngPIntkVUsHiDeb_DSM,Air_bPhysRngPIntkVUsLoDeb_DSM,Air_bPlsPIntkVUsMaxDeb_DSM,Air_bPlsPIntkVUsMinDeb_DSM
  cmp_{1..14} (14 alike) : UnitTest_Lib/RoughlyEqual  slope=0.1
  result_tws : ToWorkspace  VariableName=spec_result_001
  tws_1 : ToWorkspace  VariableName=spec_req_001_001
  tws_10 : ToWorkspace  VariableName=spec_req_001_010
  tws_11 : ToWorkspace  VariableName=spec_req_001_011
  tws_12 : ToWorkspace  VariableName=spec_req_001_012
  tws_13 : ToWorkspace  VariableName=spec_req_001_013
  tws_14 : ToWorkspace  VariableName=spec_req_001_014
  tws_2 : ToWorkspace  VariableName=spec_req_001_002
  tws_3 : ToWorkspace  VariableName=spec_req_001_003
  tws_4 : ToWorkspace  VariableName=spec_req_001_004
  tws_5 : ToWorkspace  VariableName=spec_req_001_005
  tws_6 : ToWorkspace  VariableName=spec_req_001_006
  tws_7 : ToWorkspace  VariableName=spec_req_001_007
  tws_8 : ToWorkspace  VariableName=spec_req_001_008
  tws_9 : ToWorkspace  VariableName=spec_req_001_009
  result : Outport
  wires:
  sig_Req_Bus/1 -> BS_Req/1
  sig_Result_Bus/1 -> BS_Result/1
  AndN/1 -> result/1, result_tws/1
  BS_Req/1 -> cmp_1/1  "<testSig_Air_uRawPIntkVUs>"
  BS_Result/1 -> cmp_1/2  "<Air_uRawPIntkVUs>"
  cmp_1/1 -> tws_1/1, AndN/1
  BS_Req/2 -> cmp_2/1  "<testSig_Air_pSensPIntkVUs>"
  BS_Result/2 -> cmp_2/2  "<Air_pSensPIntkVUs>"
  cmp_2/1 -> tws_2/1, AndN/2
  BS_Req/3 -> cmp_3/1  "<testSig_Air_bPIntkVUsFinalDef>"
  BS_Result/3 -> cmp_3/2  "<Air_bPIntkVUsFinalDef>"
  cmp_3/1 -> tws_3/1, AndN/3
  BS_Req/4 -> cmp_4/1  "<testSig_Air_bPIntkVUsProvDef>"
  BS_Result/4 -> cmp_4/2  "<Air_bPIntkVUsProvDef>"
  cmp_4/1 -> tws_4/1, AndN/4
  BS_Req/5 -> cmp_5/1  "<testSig_Air_bPhysRngPIntkVUsFinalDef>"
  BS_Result/5 -> cmp_5/2  "<Air_bPhysRngPIntkVUsFinalDef>"
  cmp_5/1 -> tws_5/1, AndN/5
  BS_Req/6 -> cmp_6/1  "<testSig_Air_bPhysRngPIntkVUsProvDef>"
  BS_Result/6 -> cmp_6/2  "<Air_bPhysRngPIntkVUsProvDef>"
  cmp_6/1 -> tws_6/1, AndN/6
  BS_Req/7 -> cmp_7/1  "<testSig_Air_bPlsPIntkVUsFinalDef>"
  BS_Result/7 -> cmp_7/2  "<Air_bPlsPIntkVUsFinalDef>"
  cmp_7/1 -> tws_7/1, AndN/7
  BS_Req/8 -> cmp_8/1  "<testSig_Air_bPlsPIntkVUsProvDef>"
  BS_Result/8 -> cmp_8/2  "<Air_bPlsPIntkVUsProvDef>"
  cmp_8/1 -> tws_8/1, AndN/8
  BS_Req/9 -> cmp_9/1  "<testSig_Air_bSRCPIntkVUsMaxDeb_DSM>"
  BS_Result/9 -> cmp_9/2  "<Air_bSRCPIntkVUsMaxDeb_DSM>"
  cmp_9/1 -> tws_9/1, AndN/9
  BS_Req/10 -> cmp_10/1  "<testSig_Air_bSRCPIntkVUsMinDeb_DSM>"
  BS_Result/10 -> cmp_10/2  "<Air_bSRCPIntkVUsMinDeb_DSM>"
  cmp_10/1 -> tws_10/1, AndN/10
  BS_Req/11 -> cmp_11/1  "<testSig_Air_bPhysRngPIntkVUsHiDeb_DSM>"
  BS_Result/11 -> cmp_11/2  "<Air_bPhysRngPIntkVUsHiDeb_DSM>"
  cmp_11/1 -> tws_11/1, AndN/11
  BS_Req/12 -> cmp_12/1  "<testSig_Air_bPhysRngPIntkVUsLoDeb_DSM>"
  BS_Result/12 -> cmp_12/2  "<Air_bPhysRngPIntkVUsLoDeb_DSM>"
  cmp_12/1 -> tws_12/1, AndN/12
  BS_Req/13 -> cmp_13/1  "<testSig_Air_bPlsPIntkVUsMaxDeb_DSM>"
  BS_Result/13 -> cmp_13/2  "<Air_bPlsPIntkVUsMaxDeb_DSM>"
  cmp_13/1 -> tws_13/1, AndN/13
  BS_Req/14 -> cmp_14/1  "<testSig_Air_bPlsPIntkVUsMinDeb_DSM>"
  BS_Result/14 -> cmp_14/2  "<Air_bPlsPIntkVUsMinDeb_DSM>"
  cmp_14/1 -> tws_14/1, AndN/14
